simulink model "AN_Simulink_Model_v1_fil"  (R2019b)
settings: Solver=VariableStepAuto  StartTime=0.0  StopTime=testtime  RelTol=1e-3
InitFcn:
  | AN_InitFcn_Callback
StopFcn:
  | AN_StopFcn_Callback
undefined symbols (not defined in the file or in its folder): tdres
libraries: hdlmdlgenlib x193, simulink x4, fillib x1, dspsrcs4 x1
(part 3 of 6)

== system AN_Simulink_Model_v1_fil/Auditory Nerve Model/C2 Wideband Filter/Sum7 ==
  In1 : Inport
  In2 : Inport  Port=2
  Sum7 : Sum  OutDataTypeStr=single  SampleTime=2.08333333333333e-05  SaturateOnIntegerOverflow=on  InputSameDT=on
  Out1 : Outport
  wires:
  Sum7/1 -> Out1/1
  In2/1 -> Sum7/2
  In1/1 -> Sum7/1

== system AN_Simulink_Model_v1_fil/Auditory Nerve Model/C2 Wideband Filter/Sum8 ==
  In1 : Inport
  In2 : Inport  Port=2
  Sum8 : Sum  OutDataTypeStr=single  SampleTime=2.08333333333333e-05  SaturateOnIntegerOverflow=on  InputSameDT=on
  Out1 : Outport
  wires:
  Sum8/1 -> Out1/1
  In2/1 -> Sum8/2
  In1/1 -> Sum8/1

== system AN_Simulink_Model_v1_fil/Auditory Nerve Model/C2 Wideband Filter/Sum9 ==
  In1 : Inport
  In2 : Inport  Port=2
  Sum9 : Sum  OutDataTypeStr=single  SampleTime=2.08333333333333e-05  SaturateOnIntegerOverflow=on  InputSameDT=on
  Out1 : Outport
  wires:
  Sum9/1 -> Out1/1
  In2/1 -> Sum9/2
  In1/1 -> Sum9/1

== system AN_Simulink_Model_v1_fil/Auditory Nerve Model/CP Wideband Gammatone Filter/Calculate wbout ==
  In1 : Inport  OutDataTypeStr=single  PortDimensions=1  SampleTime=2.08333333333333e-05
  In2 : Inport  Port=2  OutDataTypeStr=single  PortDimensions=1  SampleTime=2.08333333333333e-05
  Constant : Constant  Value=single(0.0007758744177408516)  OutDataTypeStr=single  SampleTime=-1
  Constant1 : Constant  Value=single(3)  OutDataTypeStr=single  SampleTime=-1
  Constant3 : Constant  Value=single(1)  OutDataTypeStr=single  SampleTime=-1
  Divide : Subsystem
      mask Display: disp('NFP\nmul');
  Divide1_to_const : Constant  Value=single(0.2)  OutDataTypeStr=single  SampleTime=-1
  Gain : Subsystem
      mask Display: disp('NFP\nmul');
  Gain_const : Constant  Value=single(10000)  OutDataTypeStr=single  SampleTime=-1
  MinMax_stage1_compare : Subsystem
      mask Display: disp('NFP\nrelop');
  MinMax_stage1_switch : Switch  Criteria=u2 ~= 0  Threshold=double(0)  OutDataTypeStr=single  SampleTime=2.08333333333333e-05
  Pow : Subsystem
      mask Display: disp('NFP\nmath2');
  Product : Subsystem
      mask Display: disp('NFP\nmul');
  Product1 : Subsystem
      mask Display: disp('NFP\nmul');
  Out1 : Outport  VectorParamsAs1DForOutWhenUnconnected=off
  wires:
  Gain/1(Out1) -> Product1/1(In1)
  MinMax_stage1_compare/1(Out1) -> MinMax_stage1_switch/2
  Product1/1(Out1) -> Out1/1
  Product/1(Out1) -> Gain/2(In2)
  Pow/1(Out1) -> Product/2(In2)
  Divide/1(Out1) -> Pow/1(In1)
  Gain_const/1 -> Gain/1(In1)
  MinMax_stage1_switch/1 -> Product1/2(In2)
  Divide1_to_const/1 -> MinMax_stage1_switch/1, MinMax_stage1_compare/2(In2)
  Constant3/1 -> MinMax_stage1_switch/3, MinMax_stage1_compare/1(In1)
  Constant1/1 -> Pow/2(In2)
  Constant/1 -> Divide/2(In2)
  In2/1 -> Divide/1(In1)
  In1/1 -> Product/1(In1)

== system AN_Simulink_Model_v1_fil/Auditory Nerve Model/CP Wideband Gammatone Filter/Gain_unaryminus ==
  In1 : Inport
  Gain_unaryminus : UnaryMinus  SampleTime=2.08333333333333e-05
  Out1 : Outport
  wires:
  Gain_unaryminus/1 -> Out1/1
  In1/1 -> Gain_unaryminus/1

== system AN_Simulink_Model_v1_fil/Auditory Nerve Model/CP Wideband Gammatone Filter/MATLAB Function1 ==
  phase : Inport  OutDataTypeStr=single  PortDimensions=1  SampleTime=2.08333333333333e-05
  delta_phase : Inport  Port=2  OutDataTypeStr=single  PortDimensions=1  SampleTime=2.08333333333333e-05
  adder : Subsystem
      mask Display: disp('NFP\nadd');
  adder_outbuff : hdlmdlgenlib/Buffer
      settings: SourceProductName=Simulink  SourceProductBaseCode=SL
  const : Constant  Value=single(6.2831854820251465)  VectorParams1D=off  OutDataTypeStr=single  SampleTime=-1
  const1 : Constant  Value=single(-6.2831854820251465)  VectorParams1D=off  OutDataTypeStr=single  SampleTime=-1
  relop : Subsystem
      mask Display: disp('NFP\nrelop');
  relop_outbuff : hdlmdlgenlib/Buffer
      settings: SourceProductName=Simulink  SourceProductBaseCode=SL
  subtract : Subsystem
      mask Display: disp('NFP\nadd');
  subtract_outbuff : hdlmdlgenlib/Buffer
      settings: SourceProductName=Simulink  SourceProductBaseCode=SL
  switch : Switch  Criteria=u2 ~= 0  Threshold=double(0)  OutDataTypeStr=single  SampleTime=2.08333333333333e-05
  wbphase : Outport  VectorParamsAs1DForOutWhenUnconnected=off
  wires:
  subtract/1(Out1) -> subtract_outbuff/1
  adder/1(Out1) -> adder_outbuff/1
  relop/1(Out1) -> relop_outbuff/1
  const1/1 -> subtract/1(In1)
  const/1 -> adder/2(In2)
  subtract_outbuff/1 -> relop/2(In2)
  adder_outbuff/1 -> switch/1
  relop_outbuff/1 -> switch/2
  switch/1 -> wbphase/1
  delta_phase/1 -> subtract/2(In2)
  phase/1 -> switch/3, relop/1(In1), adder/1(In1)

== system AN_Simulink_Model_v1_fil/Auditory Nerve Model/CP Wideband Gammatone Filter/Product ==
  In1 : Inport
  In2 : Inport  Port=2
  Product : Product  Inputs=**  OutDataTypeStr=single  SampleTime=2.08333333333333e-05
  Out1 : Outport
  wires:
  Product/1 -> Out1/1
  In2/1 -> Product/2
  In1/1 -> Product/1

== system AN_Simulink_Model_v1_fil/Auditory Nerve Model/CP Wideband Gammatone Filter/Product1 ==
  In1 : Inport
  In2 : Inport  Port=2
  Product1 : Product  Inputs=**  OutDataTypeStr=single  SampleTime=2.08333333333333e-05
  Out1 : Outport
  wires:
  Product1/1 -> Out1/1
  In2/1 -> Product1/2
  In1/1 -> Product1/1

== system AN_Simulink_Model_v1_fil/Auditory Nerve Model/CP Wideband Gammatone Filter/Product11 ==
  In1 : Inport
  In2 : Inport  Port=2
  Product11 : Product  Inputs=**  OutDataTypeStr=single  SampleTime=2.08333333333333e-05
  Out1 : Outport
  wires:
  Product11/1 -> Out1/1
  In2/1 -> Product11/2
  In1/1 -> Product11/1

== system AN_Simulink_Model_v1_fil/Auditory Nerve Model/CP Wideband Gammatone Filter/Product12 ==
  In1 : Inport
  In2 : Inport  Port=2
  Product12 : Product  Inputs=**  OutDataTypeStr=single  SampleTime=2.08333333333333e-05
  Out1 : Outport
  wires:
  Product12/1 -> Out1/1
  In2/1 -> Product12/2
  In1/1 -> Product12/1

== system AN_Simulink_Model_v1_fil/Auditory Nerve Model/CP Wideband Gammatone Filter/Product13 ==
  In1 : Inport
  In2 : Inport  Port=2
  Product13 : Product  Inputs=**  OutDataTypeStr=single  SampleTime=2.08333333333333e-05
  Out1 : Outport
  wires:
  Product13/1 -> Out1/1
  In2/1 -> Product13/2
  In1/1 -> Product13/1

== system AN_Simulink_Model_v1_fil/Auditory Nerve Model/CP Wideband Gammatone Filter/Product14 ==
  In1 : Inport
  In2 : Inport  Port=2
  Product14 : Product  Inputs=**  OutDataTypeStr=single  SampleTime=2.08333333333333e-05
  Out1 : Outport
  wires:
  Product14/1 -> Out1/1
  In2/1 -> Product14/2
  In1/1 -> Product14/1

== system AN_Simulink_Model_v1_fil/Auditory Nerve Model/CP Wideband Gammatone Filter/Product1_AC_minus_BD ==
  In1 : Inport
  In2 : Inport  Port=2
  Product1_AC_minus_BD : Sum  Inputs=+-  OutDataTypeStr=single  SampleTime=2.08333333333333e-05  SaturateOnIntegerOverflow=on  InputSameDT=on
  Out1 : Outport
  wires:
  Product1_AC_minus_BD/1 -> Out1/1
  In2/1 -> Product1_AC_minus_BD/2
  In1/1 -> Product1_AC_minus_BD/1

== system AN_Simulink_Model_v1_fil/Auditory Nerve Model/CP Wideband Gammatone Filter/Product1_AD_plus_BC ==
  In1 : Inport
  In2 : Inport  Port=2
  Product1_AD_plus_BC : Sum  OutDataTypeStr=single  SampleTime=2.08333333333333e-05  SaturateOnIntegerOverflow=on  InputSameDT=on
  Out1 : Outport
  wires:
  Product1_AD_plus_BC/1 -> Out1/1
  In2/1 -> Product1_AD_plus_BC/2
  In1/1 -> Product1_AD_plus_BC/1

== system AN_Simulink_Model_v1_fil/Auditory Nerve Model/CP Wideband Gammatone Filter/Sum ==
  In1 : Inport
  In2 : Inport  Port=2
  Sum : Sum  OutDataTypeStr=single  SampleTime=2.08333333333333e-05  SaturateOnIntegerOverflow=on  InputSameDT=on
  Out1 : Outport
  wires:
  Sum/1 -> Out1/1
  In2/1 -> Sum/2
  In1/1 -> Sum/1

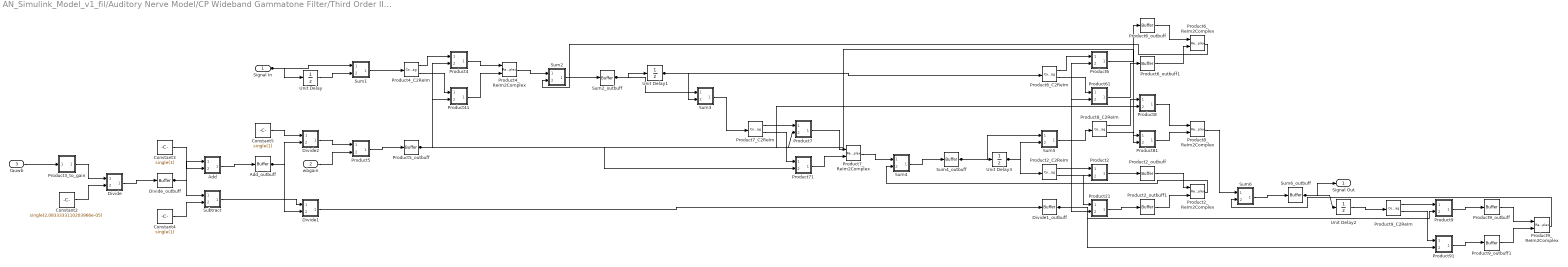
== system AN_Simulink_Model_v1_fil/Auditory Nerve Model/CP Wideband Gammatone Filter/Third Order IIR Filter ==
  Signal In : Inport  OutDataTypeStr=single  PortDimensions=1  SampleTime=2.08333333333333e-05
      settings: SignalType=complex
  wbgain : Inport  Port=2  OutDataTypeStr=single  PortDimensions=1  SampleTime=2.08333333333333e-05
  tauwb : Inport  Port=3  OutDataTypeStr=single  PortDimensions=1  SampleTime=2.08333333333333e-05
  Add : Subsystem
      mask Display: disp('NFP\nadd');
  Add_outbuff : hdlmdlgenlib/Buffer
      settings: SourceProductName=Simulink  SourceProductBaseCode=SL
  Constant2 : Constant  Value=single(2.0833333110203966e-05)  OutDataTypeStr=single  SampleTime=-1
  Constant3 : Constant  Value=single(1)  OutDataTypeStr=single  SampleTime=-1
  Constant4 : Constant  Value=single(1)  OutDataTypeStr=single  SampleTime=-1
  Constant5 : Constant  Value=single(1)  OutDataTypeStr=single  SampleTime=-1
  Divide : Subsystem
      mask Display: disp('NFP\nmul');
  Divide1 : Subsystem
      mask Display: disp('NFP\nmul');
  Divide1_outbuff : hdlmdlgenlib/Buffer
      settings: SourceProductName=Simulink  SourceProductBaseCode=SL
  Divide2 : Subsystem
      mask Display: disp('NFP\nmul');
  Divide_outbuff : hdlmdlgenlib/Buffer
      settings: SourceProductName=Simulink  SourceProductBaseCode=SL
  Product2 : Subsystem
      mask Display: disp('NFP\nmul');
  Product21 : Subsystem
      mask Display: disp('NFP\nmul');
  Product2_C2ReIm : ComplexToRealImag  SampleTime=2.08333333333333e-05
  Product2_ReIm2Complex : RealImagToComplex  SampleTime=2.08333333333333e-05
  Product2_outbuff : hdlmdlgenlib/Buffer
      settings: SourceProductName=Simulink  SourceProductBaseCode=SL
  Product2_outbuff1 : hdlmdlgenlib/Buffer
      settings: SourceProductName=Simulink  SourceProductBaseCode=SL
  Product3_to_gain : Subsystem
      mask Display: disp('NFP\ngain_pow2');
  Product4 : Subsystem
      mask Display: disp('NFP\nmul');
  Product41 : Subsystem
      mask Display: disp('NFP\nmul');
  Product4_C2ReIm : ComplexToRealImag  SampleTime=2.08333333333333e-05
  Product4_ReIm2Complex : RealImagToComplex  SampleTime=2.08333333333333e-05
  Product5 : Subsystem
      mask Display: disp('NFP\nmul');
  Product5_outbuff : hdlmdlgenlib/Buffer
      settings: SourceProductName=Simulink  SourceProductBaseCode=SL
  Product6 : Subsystem
      mask Display: disp('NFP\nmul');
  Product61 : Subsystem
      mask Display: disp('NFP\nmul');
  Product6_C2ReIm : ComplexToRealImag  SampleTime=2.08333333333333e-05
  Product6_ReIm2Complex : RealImagToComplex  SampleTime=2.08333333333333e-05
  Product6_outbuff : hdlmdlgenlib/Buffer
      settings: SourceProductName=Simulink  SourceProductBaseCode=SL
  Product6_outbuff1 : hdlmdlgenlib/Buffer
      settings: SourceProductName=Simulink  SourceProductBaseCode=SL
  Product7 : Subsystem
      mask Display: disp('NFP\nmul');
  Product71 : Subsystem
      mask Display: disp('NFP\nmul');
  Product7_C2ReIm : ComplexToRealImag  SampleTime=2.08333333333333e-05
  Product7_ReIm2Complex : RealImagToComplex  SampleTime=2.08333333333333e-05
  Product8 : Subsystem
      mask Display: disp('NFP\nmul');
  Product81 : Subsystem
      mask Display: disp('NFP\nmul');
  Product8_C2ReIm : ComplexToRealImag  SampleTime=2.08333333333333e-05
  Product8_ReIm2Complex : RealImagToComplex  SampleTime=2.08333333333333e-05
  Product9 : Subsystem
      mask Display: disp('NFP\nmul');
  Product91 : Subsystem
      mask Display: disp('NFP\nmul');
  Product9_C2ReIm : ComplexToRealImag  SampleTime=2.08333333333333e-05
  Product9_ReIm2Complex : RealImagToComplex  SampleTime=2.08333333333333e-05
  Product9_outbuff : hdlmdlgenlib/Buffer
      settings: SourceProductName=Simulink  SourceProductBaseCode=SL
  Product9_outbuff1 : hdlmdlgenlib/Buffer
      settings: SourceProductName=Simulink  SourceProductBaseCode=SL
  Subtract : Subsystem
      mask Display: disp('NFP\nadd');
  Sum1 : Subsystem
      mask Display: disp('NFP\nadd');
  Sum2 : Subsystem
      mask Display: disp('NFP\nadd');
  Sum2_outbuff : hdlmdlgenlib/Buffer
      settings: SourceProductName=Simulink  SourceProductBaseCode=SL
  Sum3 : Subsystem
      mask Display: disp('NFP\nadd');
  Sum4 : Subsystem
      mask Display: disp('NFP\nadd');
  Sum4_outbuff : hdlmdlgenlib/Buffer
      settings: SourceProductName=Simulink  SourceProductBaseCode=SL
  Sum5 : Subsystem
      mask Display: disp('NFP\nadd');
  Sum6 : Subsystem
      mask Display: disp('NFP\nadd');
  Sum6_outbuff : hdlmdlgenlib/Buffer
      settings: SourceProductName=Simulink  SourceProductBaseCode=SL
  Unit Delay{,1..3} (4 alike) : UnitDelay  InitialCondition=single(0)  SampleTime=2.08333333333333e-05
  Signal Out : Outport  VectorParamsAs1DForOutWhenUnconnected=off
  wires:
  Product91/1(Out1) -> Product9_outbuff1/1
  Product9/1(Out1) -> Product9_outbuff/1
  Product81/1(Out1) -> Product8_ReIm2Complex/2
  Product8/1(Out1) -> Product8_ReIm2Complex/1
  Product71/1(Out1) -> Product7_ReIm2Complex/2
  Product7/1(Out1) -> Product7_ReIm2Complex/1
  Product61/1(Out1) -> Product6_outbuff1/1
  Product6/1(Out1) -> Product6_outbuff/1
  Product41/1(Out1) -> Product4_ReIm2Complex/2
  Product4/1(Out1) -> Product4_ReIm2Complex/1
  Product21/1(Out1) -> Product2_outbuff1/1
  Product2/1(Out1) -> Product2_outbuff/1
  Product3_to_gain/1(Out1) -> Divide/1(In1)
  Sum6/1(Out1) -> Sum6_outbuff/1
  Sum5/1(Out1) -> Product8_C2ReIm/1
  Sum4/1(Out1) -> Sum4_outbuff/1
  Sum3/1(Out1) -> Product7_C2ReIm/1
  Sum2/1(Out1) -> Sum2_outbuff/1
  Sum1/1(Out1) -> Product4_C2ReIm/1
  Subtract/1(Out1) -> Divide1/1(In1)
  Product5/1(Out1) -> Product5_outbuff/1
  Divide2/1(Out1) -> Product5/1(In1)
  Divide1/1(Out1) -> Divide1_outbuff/1
  Divide/1(Out1) -> Divide_outbuff/1
  Add/1(Out1) -> Add_outbuff/1
  Product9_outbuff1/1 -> Product9_ReIm2Complex/2
  Product9_outbuff/1 -> Product9_ReIm2Complex/1
  Product9_C2ReIm/2 -> Product91/1(In1)
  Product9_C2ReIm/1 -> Product9/1(In1)
  Product8_C2ReIm/2 -> Product81/1(In1)
  Product8_C2ReIm/1 -> Product8/1(In1)
  Product7_C2ReIm/2 -> Product71/1(In1)
  Product7_C2ReIm/1 -> Product7/1(In1)
  Product6_outbuff1/1 -> Product6_ReIm2Complex/2
  Product6_outbuff/1 -> Product6_ReIm2Complex/1
  Product6_C2ReIm/2 -> Product61/1(In1)
  Product6_C2ReIm/1 -> Product6/1(In1)
  Product4_C2ReIm/2 -> Product41/1(In1)
  Product4_C2ReIm/1 -> Product4/1(In1)
  Product2_outbuff1/1 -> Product2_ReIm2Complex/2
  Product2_outbuff/1 -> Product2_ReIm2Complex/1
  Product2_C2ReIm/2 -> Product21/1(In1)
  Product2_C2ReIm/1 -> Product2/1(In1)
  Unit Delay3/1 -> Product2_C2ReIm/1, Sum5/2(In2)
  Unit Delay2/1 -> Product9_C2ReIm/1
  Unit Delay1/1 -> Product6_C2ReIm/1, Sum3/2(In2)
  Unit Delay/1 -> Sum1/2(In2)
  Sum6_outbuff/1 -> Signal Out/1, Unit Delay2/1
  Sum4_outbuff/1 -> Unit Delay3/1, Sum5/1(In1)
  Sum2_outbuff/1 -> Unit Delay1/1, Sum3/1(In1)
  Product9_ReIm2Complex/1 -> Sum6/2(In2)
  Product8_ReIm2Complex/1 -> Sum6/1(In1)
  Product7_ReIm2Complex/1 -> Sum4/1(In1)
  Product6_ReIm2Complex/1 -> Sum2/2(In2)
  Product5_outbuff/1 -> Product4/2(In2), Product41/2(In2), Product7/2(In2), Product71/2(In2), Product8/2(In2), Product81/2(In2)
  Product4_ReIm2Complex/1 -> Sum2/1(In1)
  Product2_ReIm2Complex/1 -> Sum4/2(In2)
  Divide1_outbuff/1 -> Product2/2(In2), Product21/2(In2), Product6/2(In2), Product61/2(In2), Product9/2(In2), Product91/2(In2)
  Divide_outbuff/1 -> Add/1(In1), Subtract/1(In1)
  Constant5/1 -> Divide2/1(In1)
  Constant4/1 -> Subtract/2(In2)
  Constant3/1 -> Add/2(In2)
  Constant2/1 -> Divide/2(In2)
  Add_outbuff/1 -> Divide1/2(In2), Divide2/2(In2)
  tauwb/1 -> Product3_to_gain/1(In1)
  wbgain/1 -> Product5/2(In2)
  Signal In/1 -> Unit Delay/1, Sum1/1(In1)

== system AN_Simulink_Model_v1_fil/Auditory Nerve Model/CP Wideband Gammatone Filter/Trigonometric Function ==
  In1 : Inport
  Trigonometric Function : Trigonometry  Operator=sincos  SampleTime=2.08333333333333e-05
  Out1 : Outport
  Out2 : Outport  Port=2
  wires:
  Trigonometric Function/2 -> Out2/1
  Trigonometric Function/1 -> Out1/1
  In1/1 -> Trigonometric Function/1

== system AN_Simulink_Model_v1_fil/Auditory Nerve Model/CP Wideband Gammatone Filter/Trigonometric Function1 ==
  In1 : Inport
  Trigonometric Function1 : Trigonometry  Operator=sincos  SampleTime=2.08333333333333e-05
  Out1 : Outport
  Out2 : Outport  Port=2
  wires:
  Trigonometric Function1/2 -> Out2/1
  Trigonometric Function1/1 -> Out1/1
  In1/1 -> Trigonometric Function1/1

== system AN_Simulink_Model_v1_fil/Auditory Nerve Model/Middle Ear Filter/Gain1_unaryminus ==
  In1 : Inport
  Gain1_unaryminus : UnaryMinus  SampleTime=2.08333333333333e-05
  Out1 : Outport
  wires:
  Gain1_unaryminus/1 -> Out1/1
  In1/1 -> Gain1_unaryminus/1

== system AN_Simulink_Model_v1_fil/Auditory Nerve Model/Middle Ear Filter/Gain2_unaryminus ==
  In1 : Inport
  Gain2_unaryminus : UnaryMinus  SampleTime=2.08333333333333e-05
  Out1 : Outport
  wires:
  Gain2_unaryminus/1 -> Out1/1
  In1/1 -> Gain2_unaryminus/1

== system AN_Simulink_Model_v1_fil/Auditory Nerve Model/Middle Ear Filter/Gain3_unaryminus ==
  In1 : Inport
  Gain3_unaryminus : UnaryMinus  SampleTime=2.08333333333333e-05
  Out1 : Outport
  wires:
  Gain3_unaryminus/1 -> Out1/1
  In1/1 -> Gain3_unaryminus/1

== system AN_Simulink_Model_v1_fil/Auditory Nerve Model/Middle Ear Filter/Gain5_unaryminus ==
  In1 : Inport
  Gain5_unaryminus : UnaryMinus  SampleTime=2.08333333333333e-05
  Out1 : Outport
  wires:
  Gain5_unaryminus/1 -> Out1/1
  In1/1 -> Gain5_unaryminus/1

== system AN_Simulink_Model_v1_fil/Auditory Nerve Model/Middle Ear Filter/Gain7_unaryminus ==
  In1 : Inport
  Gain7_unaryminus : UnaryMinus  SampleTime=2.08333333333333e-05
  Out1 : Outport
  wires:
  Gain7_unaryminus/1 -> Out1/1
  In1/1 -> Gain7_unaryminus/1

== system AN_Simulink_Model_v1_fil/Auditory Nerve Model/Middle Ear Filter/Gain8_unaryminus ==
  In1 : Inport
  Gain8_unaryminus : UnaryMinus  SampleTime=2.08333333333333e-05
  Out1 : Outport
  wires:
  Gain8_unaryminus/1 -> Out1/1
  In1/1 -> Gain8_unaryminus/1

== system AN_Simulink_Model_v1_fil/Auditory Nerve Model/Middle Ear Filter/Product ==
  In1 : Inport
  In2 : Inport  Port=2
  Product : Product  Inputs=**  OutDataTypeStr=single  SampleTime=2.08333333333333e-05
  Out1 : Outport
  wires:
  Product/1 -> Out1/1
  In2/1 -> Product/2
  In1/1 -> Product/1

== system AN_Simulink_Model_v1_fil/Auditory Nerve Model/Middle Ear Filter/Product1 ==
  In1 : Inport
  In2 : Inport  Port=2
  Product1 : Product  Inputs=**  OutDataTypeStr=single  SampleTime=2.08333333333333e-05
  Out1 : Outport
  wires:
  Product1/1 -> Out1/1
  In2/1 -> Product1/2
  In1/1 -> Product1/1

== system AN_Simulink_Model_v1_fil/Auditory Nerve Model/Middle Ear Filter/Product10 ==
  In1 : Inport
  In2 : Inport  Port=2
  Product10 : Product  Inputs=**  OutDataTypeStr=single  SampleTime=2.08333333333333e-05
  Out1 : Outport
  wires:
  Product10/1 -> Out1/1
  In2/1 -> Product10/2
  In1/1 -> Product10/1

== system AN_Simulink_Model_v1_fil/Auditory Nerve Model/Middle Ear Filter/Product11 ==
  In1 : Inport
  In2 : Inport  Port=2
  Product11 : Product  Inputs=**  OutDataTypeStr=single  SampleTime=2.08333333333333e-05
  Out1 : Outport
  wires:
  Product11/1 -> Out1/1
  In2/1 -> Product11/2
  In1/1 -> Product11/1

== system AN_Simulink_Model_v1_fil/Auditory Nerve Model/Middle Ear Filter/Product12 ==
  In1 : Inport
  In2 : Inport  Port=2
  Product12 : Product  Inputs=**  OutDataTypeStr=single  SampleTime=2.08333333333333e-05
  Out1 : Outport
  wires:
  Product12/1 -> Out1/1
  In2/1 -> Product12/2
  In1/1 -> Product12/1

== system AN_Simulink_Model_v1_fil/Auditory Nerve Model/Middle Ear Filter/Product13 ==
  In1 : Inport
  In2 : Inport  Port=2
  Product13 : Product  Inputs=**  OutDataTypeStr=single  SampleTime=2.08333333333333e-05
  Out1 : Outport
  wires:
  Product13/1 -> Out1/1
  In2/1 -> Product13/2
  In1/1 -> Product13/1

== system AN_Simulink_Model_v1_fil/Auditory Nerve Model/Middle Ear Filter/Product14 ==
  In1 : Inport
  In2 : Inport  Port=2
  Product14 : Product  Inputs=**  OutDataTypeStr=single  SampleTime=2.08333333333333e-05
  Out1 : Outport
  wires:
  Product14/1 -> Out1/1
  In2/1 -> Product14/2
  In1/1 -> Product14/1

== system AN_Simulink_Model_v1_fil/Auditory Nerve Model/Middle Ear Filter/Product15_to_gain ==
  In1 : Inport
  Product15_to_gain : Gain  Gain=single(0.5)
  Out1 : Outport
  wires:
  Product15_to_gain/1 -> Out1/1
  In1/1 -> Product15_to_gain/1

== system AN_Simulink_Model_v1_fil/Auditory Nerve Model/Middle Ear Filter/Product2 ==
  In1 : Inport
  In2 : Inport  Port=2
  Product2 : Product  Inputs=**  OutDataTypeStr=single  SampleTime=2.08333333333333e-05
  Out1 : Outport
  wires:
  Product2/1 -> Out1/1
  In2/1 -> Product2/2
  In1/1 -> Product2/1

== system AN_Simulink_Model_v1_fil/Auditory Nerve Model/Middle Ear Filter/Product3 ==
  In1 : Inport
  In2 : Inport  Port=2
  Product3 : Product  Inputs=**  OutDataTypeStr=single  SampleTime=2.08333333333333e-05
  Out1 : Outport
  wires:
  Product3/1 -> Out1/1
  In2/1 -> Product3/2
  In1/1 -> Product3/1

== system AN_Simulink_Model_v1_fil/Auditory Nerve Model/Middle Ear Filter/Product4 ==
  In1 : Inport
  In2 : Inport  Port=2
  Product4 : Product  Inputs=**  OutDataTypeStr=single  SampleTime=2.08333333333333e-05
  Out1 : Outport
  wires:
  Product4/1 -> Out1/1
  In2/1 -> Product4/2
  In1/1 -> Product4/1

== system AN_Simulink_Model_v1_fil/Auditory Nerve Model/Middle Ear Filter/Product5 ==
  In1 : Inport
  In2 : Inport  Port=2
  Product5 : Product  Inputs=**  OutDataTypeStr=single  SampleTime=2.08333333333333e-05
  Out1 : Outport
  wires:
  Product5/1 -> Out1/1
  In2/1 -> Product5/2
  In1/1 -> Product5/1

== system AN_Simulink_Model_v1_fil/Auditory Nerve Model/Middle Ear Filter/Product6 ==
  In1 : Inport
  In2 : Inport  Port=2
  Product6 : Product  Inputs=**  OutDataTypeStr=single  SampleTime=2.08333333333333e-05
  Out1 : Outport
  wires:
  Product6/1 -> Out1/1
  In2/1 -> Product6/2
  In1/1 -> Product6/1

== system AN_Simulink_Model_v1_fil/Auditory Nerve Model/Middle Ear Filter/Product7 ==
  In1 : Inport
  In2 : Inport  Port=2
  Product7 : Product  Inputs=**  OutDataTypeStr=single  SampleTime=2.08333333333333e-05
  Out1 : Outport
  wires:
  Product7/1 -> Out1/1
  In2/1 -> Product7/2
  In1/1 -> Product7/1

== system AN_Simulink_Model_v1_fil/Auditory Nerve Model/Middle Ear Filter/Product8 ==
  In1 : Inport
  In2 : Inport  Port=2
  Product8 : Product  Inputs=**  OutDataTypeStr=single  SampleTime=2.08333333333333e-05
  Out1 : Outport
  wires:
  Product8/1 -> Out1/1
  In2/1 -> Product8/2
  In1/1 -> Product8/1

== system AN_Simulink_Model_v1_fil/Auditory Nerve Model/Middle Ear Filter/Product9 ==
  In1 : Inport
  In2 : Inport  Port=2
  Product9 : Product  Inputs=**  OutDataTypeStr=single  SampleTime=2.08333333333333e-05
  Out1 : Outport
  wires:
  Product9/1 -> Out1/1
  In2/1 -> Product9/2
  In1/1 -> Product9/1

== system AN_Simulink_Model_v1_fil/Auditory Nerve Model/Middle Ear Filter/Sum ==
  In1 : Inport
  In2 : Inport  Port=2
  Sum : Sum  OutDataTypeStr=single  SampleTime=2.08333333333333e-05  SaturateOnIntegerOverflow=on  InputSameDT=on
  Out1 : Outport
  wires:
  Sum/1 -> Out1/1
  In2/1 -> Sum/2
  In1/1 -> Sum/1

== system AN_Simulink_Model_v1_fil/Auditory Nerve Model/Middle Ear Filter/Sum1 ==
  In1 : Inport
  In2 : Inport  Port=2
  Sum1 : Sum  OutDataTypeStr=single  SampleTime=2.08333333333333e-05  SaturateOnIntegerOverflow=on  InputSameDT=on
  Out1 : Outport
  wires:
  Sum1/1 -> Out1/1
  In2/1 -> Sum1/2
  In1/1 -> Sum1/1

== system AN_Simulink_Model_v1_fil/Auditory Nerve Model/Middle Ear Filter/Sum10 ==
  In1 : Inport
  In2 : Inport  Port=2
  Sum10 : Sum  OutDataTypeStr=single  SampleTime=2.08333333333333e-05  SaturateOnIntegerOverflow=on  InputSameDT=on
  Out1 : Outport
  wires:
  Sum10/1 -> Out1/1
  In2/1 -> Sum10/2
  In1/1 -> Sum10/1

== system AN_Simulink_Model_v1_fil/Auditory Nerve Model/Middle Ear Filter/Sum11 ==
  In1 : Inport
  In2 : Inport  Port=2
  Sum11 : Sum  OutDataTypeStr=single  SampleTime=2.08333333333333e-05  SaturateOnIntegerOverflow=on  InputSameDT=on
  Out1 : Outport
  wires:
  Sum11/1 -> Out1/1
  In2/1 -> Sum11/2
  In1/1 -> Sum11/1

== system AN_Simulink_Model_v1_fil/Auditory Nerve Model/Middle Ear Filter/Sum2 ==
  In1 : Inport
  In2 : Inport  Port=2
  Sum2 : Sum  OutDataTypeStr=single  SampleTime=2.08333333333333e-05  SaturateOnIntegerOverflow=on  InputSameDT=on
  Out1 : Outport
  wires:
  Sum2/1 -> Out1/1
  In2/1 -> Sum2/2
  In1/1 -> Sum2/1

== system AN_Simulink_Model_v1_fil/Auditory Nerve Model/Middle Ear Filter/Sum3 ==
  In1 : Inport
  In2 : Inport  Port=2
  Sum3 : Sum  OutDataTypeStr=single  SampleTime=2.08333333333333e-05  SaturateOnIntegerOverflow=on  InputSameDT=on
  Out1 : Outport
  wires:
  Sum3/1 -> Out1/1
  In2/1 -> Sum3/2
  In1/1 -> Sum3/1

== system AN_Simulink_Model_v1_fil/Auditory Nerve Model/Middle Ear Filter/Sum4 ==
  In1 : Inport
  In2 : Inport  Port=2
  Sum4 : Sum  OutDataTypeStr=single  SampleTime=2.08333333333333e-05  SaturateOnIntegerOverflow=on  InputSameDT=on
  Out1 : Outport
  wires:
  Sum4/1 -> Out1/1
  In2/1 -> Sum4/2
  In1/1 -> Sum4/1

== system AN_Simulink_Model_v1_fil/Auditory Nerve Model/Middle Ear Filter/Sum5 ==
  In1 : Inport
  In2 : Inport  Port=2
  Sum5 : Sum  OutDataTypeStr=single  SampleTime=2.08333333333333e-05  SaturateOnIntegerOverflow=on  InputSameDT=on
  Out1 : Outport
  wires:
  Sum5/1 -> Out1/1
  In2/1 -> Sum5/2
  In1/1 -> Sum5/1

== system AN_Simulink_Model_v1_fil/Auditory Nerve Model/Middle Ear Filter/Sum6 ==
  In1 : Inport
  In2 : Inport  Port=2
  Sum6 : Sum  OutDataTypeStr=single  SampleTime=2.08333333333333e-05  SaturateOnIntegerOverflow=on  InputSameDT=on
  Out1 : Outport
  wires:
  Sum6/1 -> Out1/1
  In2/1 -> Sum6/2
  In1/1 -> Sum6/1

== system AN_Simulink_Model_v1_fil/Auditory Nerve Model/Middle Ear Filter/Sum7 ==
  In1 : Inport
  In2 : Inport  Port=2
  Sum7 : Sum  OutDataTypeStr=single  SampleTime=2.08333333333333e-05  SaturateOnIntegerOverflow=on  InputSameDT=on
  Out1 : Outport
  wires:
  Sum7/1 -> Out1/1
  In2/1 -> Sum7/2
  In1/1 -> Sum7/1

== system AN_Simulink_Model_v1_fil/Auditory Nerve Model/Middle Ear Filter/Sum8 ==
  In1 : Inport
  In2 : Inport  Port=2
  Sum8 : Sum  OutDataTypeStr=single  SampleTime=2.08333333333333e-05  SaturateOnIntegerOverflow=on  InputSameDT=on
  Out1 : Outport
  wires:
  Sum8/1 -> Out1/1
  In2/1 -> Sum8/2
  In1/1 -> Sum8/1

== system AN_Simulink_Model_v1_fil/Auditory Nerve Model/Middle Ear Filter/Sum9 ==
  In1 : Inport
  In2 : Inport  Port=2
  Sum9 : Sum  OutDataTypeStr=single  SampleTime=2.08333333333333e-05  SaturateOnIntegerOverflow=on  InputSameDT=on
  Out1 : Outport
  wires:
  Sum9/1 -> Out1/1
  In2/1 -> Sum9/2
  In1/1 -> Sum9/1

== system AN_Simulink_Model_v1_fil/Auditory Nerve Model/Subsystem/IHC C1 NL Logarithmic Function ==
  stimulus : Inport  OutDataTypeStr=single  PortDimensions=1  SampleTime=2.08333333333333e-05
  Abs1 : Subsystem
      mask Display: disp('NFP\nabs');
  Add1 : Subsystem
      mask Display: disp('NFP\nadd');
  Compare To Zero1_const : Constant  Value=single(0)  OutDataTypeStr=single  SampleTime=-1
  Compare To Zero1_relop : Subsystem
      mask Display: disp('NFP\nrelop');
  Compare To Zero1_relop_outbuff : hdlmdlgenlib/Buffer
      settings: SourceProductName=Simulink  SourceProductBaseCode=SL
  Constant1 : Constant  Value=single(2000)  OutDataTypeStr=single  SampleTime=-1
  Constant2 : Constant  Value=single(1)  OutDataTypeStr=single  SampleTime=-1
  Constant3 : Constant  Value=single(0.1)  OutDataTypeStr=single  SampleTime=-1
  Log1 : Subsystem
      mask Display: disp('NFP\nmath');
  Product3 : Subsystem
      mask Display: disp('NFP\nmul');
  Product4 : Subsystem
      mask Display: disp('NFP\nmul');
  Product4_outbuff : hdlmdlgenlib/Buffer
      settings: SourceProductName=Simulink  SourceProductBaseCode=SL
  Subsystem1 : Subsystem
  Switch1 : Switch  Criteria=u2 ~= 0  Threshold=double(0)  OutDataTypeStr=single  SampleTime=2.08333333333333e-05
  output : Outport  VectorParamsAs1DForOutWhenUnconnected=off
  wires:
  Product4/1(Out1) -> Product4_outbuff/1
  Product3/1(Out1) -> Add1/1(In1)
  Log1/1(Out1) -> Product4/1(In1)
  Compare To Zero1_relop/1(Out1) -> Compare To Zero1_relop_outbuff/1
  Add1/1(Out1) -> Log1/1(In1)
  Abs1/1(Out1) -> Product3/1(In1)
  Compare To Zero1_const/1 -> Compare To Zero1_relop/2(In2)
  Switch1/1 -> output/1
  Subsystem1/1(Out1) -> Switch1/1
  Product4_outbuff/1 -> Subsystem1/2(In2), Switch1/3
  Constant3/1 -> Product4/2(In2)
  Constant2/1 -> Add1/2(In2)
  Constant1/1 -> Product3/2(In2)
  Compare To Zero1_relop_outbuff/1 -> Subsystem1/3(Enable), Switch1/2
  stimulus/1 -> Subsystem1/1(x), Abs1/1(In1), Compare To Zero1_relop/1(In1)

== system AN_Simulink_Model_v1_fil/Auditory Nerve Model/Subsystem/IHC C2 NL Logarithmic Function ==
  stimulus : Inport  OutDataTypeStr=single  PortDimensions=1  SampleTime=2.08333333333333e-05
  Abs1 : Subsystem
      mask Display: disp('NFP\nabs');
  Add1 : Subsystem
      mask Display: disp('NFP\nadd');
  Compare To Zero1_const : Constant  Value=single(0)  OutDataTypeStr=single  SampleTime=-1
  Compare To Zero1_relop : Subsystem
      mask Display: disp('NFP\nrelop');
  Compare To Zero1_relop_outbuff : hdlmdlgenlib/Buffer
      settings: SourceProductName=Simulink  SourceProductBaseCode=SL
  Constant1 : Constant  Value=single(2000)  OutDataTypeStr=single  SampleTime=-1
  Constant2 : Constant  Value=single(1)  OutDataTypeStr=single  SampleTime=-1
  Constant3 : Constant  Value=single(0.2)  OutDataTypeStr=single  SampleTime=-1
  Log1 : Subsystem
      mask Display: disp('NFP\nmath');
  Product3 : Subsystem
      mask Display: disp('NFP\nmul');
  Product4 : Subsystem
      mask Display: disp('NFP\nmul');
  Product4_outbuff : hdlmdlgenlib/Buffer
      settings: SourceProductName=Simulink  SourceProductBaseCode=SL
  Subsystem1 : Subsystem
  Switch1 : Switch  Criteria=u2 ~= 0  Threshold=double(0)  OutDataTypeStr=single  SampleTime=2.08333333333333e-05
  output : Outport  VectorParamsAs1DForOutWhenUnconnected=off
  wires:
  Product4/1(Out1) -> Product4_outbuff/1
  Product3/1(Out1) -> Add1/1(In1)
  Log1/1(Out1) -> Product4/1(In1)
  Compare To Zero1_relop/1(Out1) -> Compare To Zero1_relop_outbuff/1
  Add1/1(Out1) -> Log1/1(In1)
  Abs1/1(Out1) -> Product3/1(In1)
  Compare To Zero1_const/1 -> Compare To Zero1_relop/2(In2)
  Switch1/1 -> output/1
  Subsystem1/1(Out1) -> Switch1/1
  Product4_outbuff/1 -> Subsystem1/2(In2), Switch1/3
  Constant3/1 -> Product4/2(In2)
  Constant2/1 -> Add1/2(In2)
  Constant1/1 -> Product3/2(In2)
  Compare To Zero1_relop_outbuff/1 -> Subsystem1/3(Enable), Switch1/2
  stimulus/1 -> Subsystem1/1(x), Abs1/1(In1), Compare To Zero1_relop/1(In1)

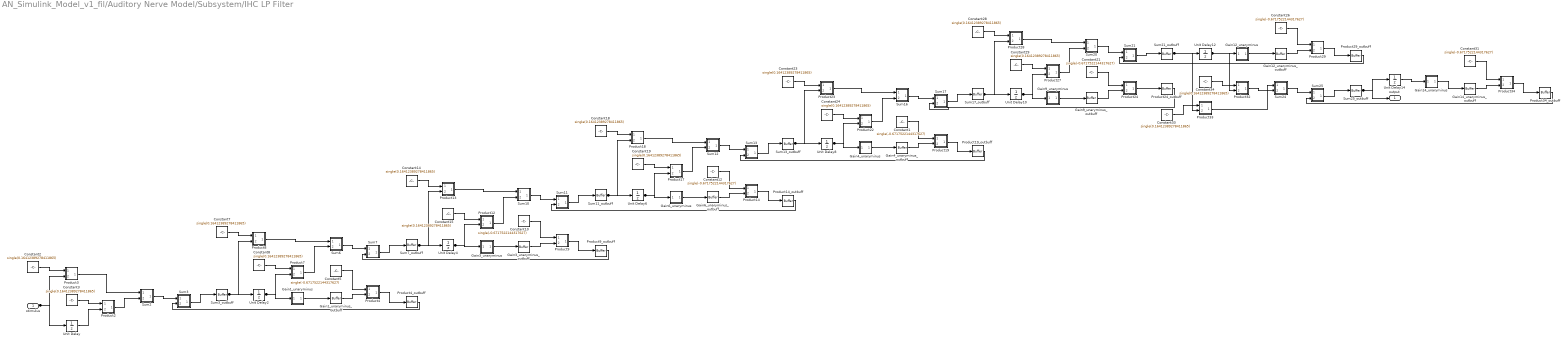
== system AN_Simulink_Model_v1_fil/Auditory Nerve Model/Subsystem/IHC LP Filter ==
  stimulus : Inport  OutDataTypeStr=single  PortDimensions=1  SampleTime=2.08333333333333e-05
  Constant{1,5,10,12,21,26,31} (7 alike) : Constant  Value=single(-0.6717522144317627)  OutDataTypeStr=single  SampleTime=-1
  Constant{2..3,7..8,14..15,18..19,23..24,28..29,33..34} (14 alike) : Constant  Value=single(0.16412389278411865)  OutDataTypeStr=single  SampleTime=-1
  Gain12_unaryminus : Subsystem
      mask Display: disp('NFP\numinus');
  Gain12_unaryminus_outbuff : hdlmdlgenlib/Buffer
      settings: SourceProductName=Simulink  SourceProductBaseCode=SL
  Gain14_unaryminus : Subsystem
      mask Display: disp('NFP\numinus');
  Gain14_unaryminus_outbuff : hdlmdlgenlib/Buffer
      settings: SourceProductName=Simulink  SourceProductBaseCode=SL
  Gain1_unaryminus : Subsystem
      mask Display: disp('NFP\numinus');
  Gain1_unaryminus_outbuff : hdlmdlgenlib/Buffer
      settings: SourceProductName=Simulink  SourceProductBaseCode=SL
  Gain3_unaryminus : Subsystem
      mask Display: disp('NFP\numinus');
  Gain3_unaryminus_outbuff : hdlmdlgenlib/Buffer
      settings: SourceProductName=Simulink  SourceProductBaseCode=SL
  Gain4_unaryminus : Subsystem
      mask Display: disp('NFP\numinus');
  Gain4_unaryminus_outbuff : hdlmdlgenlib/Buffer
      settings: SourceProductName=Simulink  SourceProductBaseCode=SL
  Gain6_unaryminus : Subsystem
      mask Display: disp('NFP\numinus');
  Gain6_unaryminus_outbuff : hdlmdlgenlib/Buffer
      settings: SourceProductName=Simulink  SourceProductBaseCode=SL
  Gain9_unaryminus : Subsystem
      mask Display: disp('NFP\numinus');
  Gain9_unaryminus_outbuff : hdlmdlgenlib/Buffer
      settings: SourceProductName=Simulink  SourceProductBaseCode=SL
  Product12 : Subsystem
      mask Display: disp('NFP\nmul');
  Product13 : Subsystem
      mask Display: disp('NFP\nmul');
  Product14 : Subsystem
      mask Display: disp('NFP\nmul');
  Product14_outbuff : hdlmdlgenlib/Buffer
      settings: SourceProductName=Simulink  SourceProductBaseCode=SL
  Product17 : Subsystem
      mask Display: disp('NFP\nmul');
  Product18 : Subsystem
      mask Display: disp('NFP\nmul');
  Product19 : Subsystem
      mask Display: disp('NFP\nmul');
  Product19_outbuff : hdlmdlgenlib/Buffer
      settings: SourceProductName=Simulink  SourceProductBaseCode=SL
  Product2 : Subsystem
      mask Display: disp('NFP\nmul');
  Product22 : Subsystem
      mask Display: disp('NFP\nmul');
  Product23 : Subsystem
      mask Display: disp('NFP\nmul');
  Product24 : Subsystem
      mask Display: disp('NFP\nmul');
  Product24_outbuff : hdlmdlgenlib/Buffer
      settings: SourceProductName=Simulink  SourceProductBaseCode=SL
  Product27 : Subsystem
      mask Display: disp('NFP\nmul');
  Product28 : Subsystem
      mask Display: disp('NFP\nmul');
  Product29 : Subsystem
      mask Display: disp('NFP\nmul');
  Product29_outbuff : hdlmdlgenlib/Buffer
      settings: SourceProductName=Simulink  SourceProductBaseCode=SL
  Product3 : Subsystem
      mask Display: disp('NFP\nmul');
  Product32 : Subsystem
      mask Display: disp('NFP\nmul');
  Product33 : Subsystem
      mask Display: disp('NFP\nmul');
  Product34 : Subsystem
      mask Display: disp('NFP\nmul');
  Product34_outbuff : hdlmdlgenlib/Buffer
      settings: SourceProductName=Simulink  SourceProductBaseCode=SL
  Product4 : Subsystem
      mask Display: disp('NFP\nmul');
  Product4_outbuff : hdlmdlgenlib/Buffer
      settings: SourceProductName=Simulink  SourceProductBaseCode=SL
  Product7 : Subsystem
      mask Display: disp('NFP\nmul');
  Product8 : Subsystem
      mask Display: disp('NFP\nmul');
  Product9 : Subsystem
      mask Display: disp('NFP\nmul');
  Product9_outbuff : hdlmdlgenlib/Buffer
      settings: SourceProductName=Simulink  SourceProductBaseCode=SL
  Sum10 : Subsystem
      mask Display: disp('NFP\nadd');
  Sum11 : Subsystem
      mask Display: disp('NFP\nadd');
  Sum11_outbuff : hdlmdlgenlib/Buffer
      settings: SourceProductName=Simulink  SourceProductBaseCode=SL
  Sum12 : Subsystem
      mask Display: disp('NFP\nadd');
  Sum13 : Subsystem
      mask Display: disp('NFP\nadd');
  Sum13_outbuff : hdlmdlgenlib/Buffer
      settings: SourceProductName=Simulink  SourceProductBaseCode=SL
  Sum16 : Subsystem
      mask Display: disp('NFP\nadd');
  Sum17 : Subsystem
      mask Display: disp('NFP\nadd');
  Sum17_outbuff : hdlmdlgenlib/Buffer
      settings: SourceProductName=Simulink  SourceProductBaseCode=SL
  Sum2 : Subsystem
      mask Display: disp('NFP\nadd');
  Sum20 : Subsystem
      mask Display: disp('NFP\nadd');
  Sum21 : Subsystem
      mask Display: disp('NFP\nadd');
  Sum21_outbuff : hdlmdlgenlib/Buffer
      settings: SourceProductName=Simulink  SourceProductBaseCode=SL
  Sum24 : Subsystem
      mask Display: disp('NFP\nadd');
  Sum25 : Subsystem
      mask Display: disp('NFP\nadd');
  Sum25_outbuff : hdlmdlgenlib/Buffer
      settings: SourceProductName=Simulink  SourceProductBaseCode=SL
  Sum3 : Subsystem
      mask Display: disp('NFP\nadd');
  Sum3_outbuff : hdlmdlgenlib/Buffer
      settings: SourceProductName=Simulink  SourceProductBaseCode=SL
  Sum6 : Subsystem
      mask Display: disp('NFP\nadd');
  Sum7 : Subsystem
      mask Display: disp('NFP\nadd');
  Sum7_outbuff : hdlmdlgenlib/Buffer
      settings: SourceProductName=Simulink  SourceProductBaseCode=SL
  Unit Delay{,2,4,6,8,10,12,14} (8 alike) : UnitDelay  InitialCondition=single(0)  SampleTime=2.08333333333333e-05
  output : Outport  VectorParamsAs1DForOutWhenUnconnected=off
  wires:
  Sum7/1(Out1) -> Sum7_outbuff/1
  Sum6/1(Out1) -> Sum7/1(In1)
  Sum3/1(Out1) -> Sum3_outbuff/1
  Sum25/1(Out1) -> Sum25_outbuff/1
  Sum24/1(Out1) -> Sum25/1(In1)
  Sum21/1(Out1) -> Sum21_outbuff/1
  Sum20/1(Out1) -> Sum21/1(In1)
  Sum2/1(Out1) -> Sum3/1(In1)
  Sum17/1(Out1) -> Sum17_outbuff/1
  Sum16/1(Out1) -> Sum17/1(In1)
  Sum13/1(Out1) -> Sum13_outbuff/1
  Sum12/1(Out1) -> Sum13/1(In1)
  Sum11/1(Out1) -> Sum11_outbuff/1
  Sum10/1(Out1) -> Sum11/1(In1)
  Product9/1(Out1) -> Product9_outbuff/1
  Product8/1(Out1) -> Sum6/1(In1)
  Product7/1(Out1) -> Sum6/2(In2)
  Product4/1(Out1) -> Product4_outbuff/1
  Product34/1(Out1) -> Product34_outbuff/1
  Product33/1(Out1) -> Sum24/1(In1)
  Product32/1(Out1) -> Sum24/2(In2)
  Product3/1(Out1) -> Sum2/1(In1)
  Product29/1(Out1) -> Product29_outbuff/1
  Product28/1(Out1) -> Sum20/1(In1)
  Product27/1(Out1) -> Sum20/2(In2)
  Product24/1(Out1) -> Product24_outbuff/1
  Product23/1(Out1) -> Sum16/1(In1)
  Product22/1(Out1) -> Sum16/2(In2)
  Product2/1(Out1) -> Sum2/2(In2)
  Product19/1(Out1) -> Product19_outbuff/1
  Product18/1(Out1) -> Sum12/1(In1)
  Product17/1(Out1) -> Sum12/2(In2)
  Product14/1(Out1) -> Product14_outbuff/1
  Product13/1(Out1) -> Sum10/1(In1)
  Product12/1(Out1) -> Sum10/2(In2)
  Gain9_unaryminus/1(Out1) -> Gain9_unaryminus_outbuff/1
  Gain6_unaryminus/1(Out1) -> Gain6_unaryminus_outbuff/1
  Gain4_unaryminus/1(Out1) -> Gain4_unaryminus_outbuff/1
  Gain3_unaryminus/1(Out1) -> Gain3_unaryminus_outbuff/1
  Gain14_unaryminus/1(Out1) -> Gain14_unaryminus_outbuff/1
  Gain12_unaryminus/1(Out1) -> Gain12_unaryminus_outbuff/1
  Gain1_unaryminus/1(Out1) -> Gain1_unaryminus_outbuff/1
  Unit Delay8/1 -> Gain4_unaryminus/1(In1), Product22/2(In2)
  Unit Delay6/1 -> Gain6_unaryminus/1(In1), Product17/2(In2)
  Unit Delay4/1 -> Gain3_unaryminus/1(In1), Product12/2(In2)
  Unit Delay2/1 -> Gain1_unaryminus/1(In1), Product7/2(In2)
  Unit Delay14/1 -> Gain14_unaryminus/1(In1)
  Unit Delay12/1 -> Gain12_unaryminus/1(In1), Product32/2(In2)
  Unit Delay10/1 -> Gain9_unaryminus/1(In1), Product27/2(In2)
  Unit Delay/1 -> Product2/2(In2)
  Sum7_outbuff/1 -> Unit Delay4/1, Product13/2(In2)
  Sum3_outbuff/1 -> Unit Delay2/1, Product8/2(In2)
  Sum25_outbuff/1 -> output/1, Unit Delay14/1
  Sum21_outbuff/1 -> Unit Delay12/1, Product33/2(In2)
  Sum17_outbuff/1 -> Unit Delay10/1, Product28/2(In2)
  Sum13_outbuff/1 -> Unit Delay8/1, Product23/2(In2)
  Sum11_outbuff/1 -> Unit Delay6/1, Product18/2(In2)
  Product9_outbuff/1 -> Sum7/2(In2)
  Product4_outbuff/1 -> Sum3/2(In2)
  Product34_outbuff/1 -> Sum25/2(In2)
  Product29_outbuff/1 -> Sum21/2(In2)
  Product24_outbuff/1 -> Sum17/2(In2)
  Product19_outbuff/1 -> Sum13/2(In2)
  Product14_outbuff/1 -> Sum11/2(In2)
  Gain9_unaryminus_outbuff/1 -> Product24/2(In2)
  Gain6_unaryminus_outbuff/1 -> Product14/2(In2)
  Gain4_unaryminus_outbuff/1 -> Product19/2(In2)
  Gain3_unaryminus_outbuff/1 -> Product9/2(In2)
  Gain14_unaryminus_outbuff/1 -> Product34/2(In2)
  Gain12_unaryminus_outbuff/1 -> Product29/2(In2)
  Gain1_unaryminus_outbuff/1 -> Product4/2(In2)
  Constant8/1 -> Product7/1(In1)
  Constant7/1 -> Product8/1(In1)
  Constant5/1 -> Product4/1(In1)
  Constant34/1 -> Product32/1(In1)
  Constant33/1 -> Product33/1(In1)
  Constant31/1 -> Product34/1(In1)
  Constant3/1 -> Product2/1(In1)
  Constant29/1 -> Product27/1(In1)
  Constant28/1 -> Product28/1(In1)
  Constant26/1 -> Product29/1(In1)
  Constant24/1 -> Product22/1(In1)
  Constant23/1 -> Product23/1(In1)
  Constant21/1 -> Product24/1(In1)
  Constant2/1 -> Product3/1(In1)
  Constant19/1 -> Product17/1(In1)
  Constant18/1 -> Product18/1(In1)
  Constant15/1 -> Product12/1(In1)
  Constant14/1 -> Product13/1(In1)
  Constant12/1 -> Product14/1(In1)
  Constant10/1 -> Product9/1(In1)
  Constant1/1 -> Product19/1(In1)
  stimulus/1 -> Unit Delay/1, Product3/2(In2)

== system AN_Simulink_Model_v1_fil/Auditory Nerve Model/Subsystem/Sum1 ==
  In1 : Inport
  In2 : Inport  Port=2
  Sum1 : Sum  OutDataTypeStr=single  SampleTime=2.08333333333333e-05  SaturateOnIntegerOverflow=on  InputSameDT=on
  Out1 : Outport
  wires:
  Sum1/1 -> Out1/1
  In2/1 -> Sum1/2
  In1/1 -> Sum1/1

== system AN_Simulink_Model_v1_fil/Auditory Nerve Model/Subsystem1/Calculate tauc1 ==
  In1 : Inport  OutDataTypeStr=single  PortDimensions=1  SampleTime=2.08333333333333e-05
  Add : Subsystem
      mask Display: disp('NFP\nadd');
  Constant1 : Constant  Value=single(0.00046310402103699744)  OutDataTypeStr=single  SampleTime=-1
  Constant2 : Constant  Value=single(0.00046310402103699744)  OutDataTypeStr=single  SampleTime=-1
  Product_to_gain : Subsystem
      mask Display: disp('NFP\ngain_pow2');
  Subtract : Subsystem
      mask Display: disp('NFP\nadd');
  Out1 : Outport  VectorParamsAs1DForOutWhenUnconnected=off
  wires:
  Product_to_gain/1(Out1) -> Add/1(In1)
  Subtract/1(Out1) -> Product_to_gain/1(In1)
  Add/1(Out1) -> Out1/1
  Constant2/1 -> Add/2(In2)
  Constant1/1 -> Subtract/2(In2)
  In1/1 -> Subtract/1(In1)

== system AN_Simulink_Model_v1_fil/Auditory Nerve Model/Subsystem1/NL After OHC Function ==
  stimulus : Inport  OutDataTypeStr=single  PortDimensions=1  SampleTime=2.08333333333333e-05
  Abs : Subsystem
      mask Display: disp('NFP\nabs');
  Add3 : Subsystem
      mask Display: disp('NFP\nadd');
  Constant12 : Constant  Value=single(0.05)  OutDataTypeStr=single  SampleTime=-1
  Constant15 : Constant  Value=single(0.003011211520060897)  OutDataTypeStr=single  SampleTime=-1
  Constant5 : Constant  Value=single(0.146789088845253)  OutDataTypeStr=single  SampleTime=-1
  Divide1 : Subsystem
      mask Display: disp('NFP\nmul');
  Exp : Subsystem
      mask Display: disp('NFP\nmath');
  Gain2_unaryminus : Subsystem
      mask Display: disp('NFP\numinus');
  Product3 : Subsystem
      mask Display: disp('NFP\nmul');
  Product4 : Subsystem
      mask Display: disp('NFP\nmul');
  Product4_outbuff : hdlmdlgenlib/Buffer
      settings: SourceProductName=Simulink  SourceProductBaseCode=SL
  Saturation_LowerConst : Constant  Value=single(0.00046310402103699744)  OutDataTypeStr=single  SampleTime=-1
  Saturation_LowerRelop : Subsystem
      mask Display: disp('NFP\nrelop');
  Saturation_Switch1 : Switch  Criteria=u2 ~= 0  Threshold=double(0)  OutDataTypeStr=single  SampleTime=2.08333333333333e-05
  Saturation_Switch2 : Switch  Criteria=u2 ~= 0  Threshold=double(0)  OutDataTypeStr=single  SampleTime=2.08333333333333e-05
  Saturation_UpperConst : Constant  Value=single(0.003011211520060897)  OutDataTypeStr=single  SampleTime=-1
  Saturation_UpperRelop : Subsystem
      mask Display: disp('NFP\nrelop');
  Subtract4_to_const : Constant  Value=single(0.95)  OutDataTypeStr=single  SampleTime=-1
  output : Outport  VectorParamsAs1DForOutWhenUnconnected=off
  wires:
  Saturation_LowerRelop/1(Out1) -> Saturation_Switch2/2
  Saturation_UpperRelop/1(Out1) -> Saturation_Switch1/2
  Product4/1(Out1) -> Product4_outbuff/1
  Product3/1(Out1) -> Add3/2(In2)
  Exp/1(Out1) -> Product3/2(In2)
  Divide1/1(Out1) -> Gain2_unaryminus/1(In1)
  Add3/1(Out1) -> Product4/2(In2)
  Abs/1(Out1) -> Divide1/1(In1)
  Gain2_unaryminus/1(Out1) -> Exp/1(In1)
  Saturation_Switch1/1 -> Saturation_Switch2/3
  Saturation_UpperConst/1 -> Saturation_Switch2/1, Saturation_LowerRelop/2(In2)
  Saturation_LowerConst/1 -> Saturation_Switch1/1, Saturation_UpperRelop/2(In2)
  Subtract4_to_const/1 -> Product3/1(In1)
  Saturation_Switch2/1 -> output/1
  Product4_outbuff/1 -> Saturation_Switch1/3, Saturation_UpperRelop/1(In1), Saturation_LowerRelop/1(In1)
  Constant5/1 -> Divide1/2(In2)
  Constant15/1 -> Product4/1(In1)
  Constant12/1 -> Add3/1(In1)
  stimulus/1 -> Abs/1(In1)

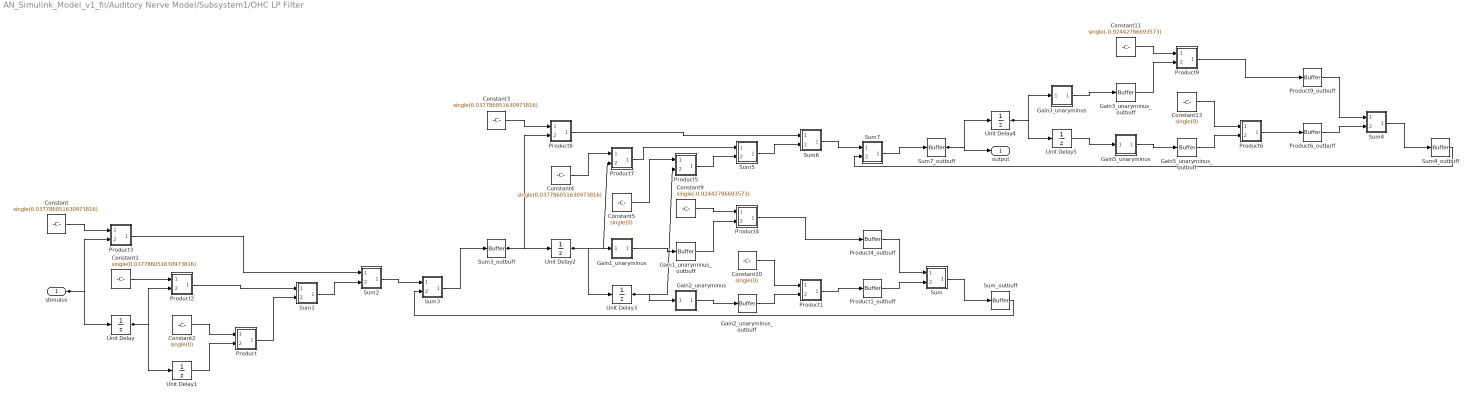
== system AN_Simulink_Model_v1_fil/Auditory Nerve Model/Subsystem1/OHC LP Filter ==
  stimulus : Inport  OutDataTypeStr=single  PortDimensions=1  SampleTime=2.08333333333333e-05
  Constant{,1,3..4} (4 alike) : Constant  Value=single(0.037786051630973816)  OutDataTypeStr=single  SampleTime=-1
  Constant{2,5,10,13} (4 alike) : Constant  Value=single(0)  OutDataTypeStr=single  SampleTime=-1
  Constant11 : Constant  Value=single(-0.92442786693573)  OutDataTypeStr=single  SampleTime=-1
  Constant9 : Constant  Value=single(-0.92442786693573)  OutDataTypeStr=single  SampleTime=-1
  Gain1_unaryminus : Subsystem
      mask Display: disp('NFP\numinus');
  Gain1_unaryminus_outbuff : hdlmdlgenlib/Buffer
      settings: SourceProductName=Simulink  SourceProductBaseCode=SL
  Gain2_unaryminus : Subsystem
      mask Display: disp('NFP\numinus');
  Gain2_unaryminus_outbuff : hdlmdlgenlib/Buffer
      settings: SourceProductName=Simulink  SourceProductBaseCode=SL
  Gain3_unaryminus : Subsystem
      mask Display: disp('NFP\numinus');
  Gain3_unaryminus_outbuff : hdlmdlgenlib/Buffer
      settings: SourceProductName=Simulink  SourceProductBaseCode=SL
  Gain5_unaryminus : Subsystem
      mask Display: disp('NFP\numinus');
  Gain5_unaryminus_outbuff : hdlmdlgenlib/Buffer
      settings: SourceProductName=Simulink  SourceProductBaseCode=SL
  Product : Subsystem
      mask Display: disp('NFP\nmul');
  Product1 : Subsystem
      mask Display: disp('NFP\nmul');
  Product1_outbuff : hdlmdlgenlib/Buffer
      settings: SourceProductName=Simulink  SourceProductBaseCode=SL
  Product2 : Subsystem
      mask Display: disp('NFP\nmul');
  Product3 : Subsystem
      mask Display: disp('NFP\nmul');
  Product4 : Subsystem
      mask Display: disp('NFP\nmul');
  Product4_outbuff : hdlmdlgenlib/Buffer
      settings: SourceProductName=Simulink  SourceProductBaseCode=SL
  Product5 : Subsystem
      mask Display: disp('NFP\nmul');
  Product6 : Subsystem
      mask Display: disp('NFP\nmul');
  Product6_outbuff : hdlmdlgenlib/Buffer
      settings: SourceProductName=Simulink  SourceProductBaseCode=SL
  Product7 : Subsystem
      mask Display: disp('NFP\nmul');
  Product8 : Subsystem
      mask Display: disp('NFP\nmul');
  Product9 : Subsystem
      mask Display: disp('NFP\nmul');
  Product9_outbuff : hdlmdlgenlib/Buffer
      settings: SourceProductName=Simulink  SourceProductBaseCode=SL
  Sum : Subsystem
      mask Display: disp('NFP\nadd');
  Sum1 : Subsystem
      mask Display: disp('NFP\nadd');
  Sum2 : Subsystem
      mask Display: disp('NFP\nadd');
  Sum3 : Subsystem
      mask Display: disp('NFP\nadd');
  Sum3_outbuff : hdlmdlgenlib/Buffer
      settings: SourceProductName=Simulink  SourceProductBaseCode=SL
  Sum4 : Subsystem
      mask Display: disp('NFP\nadd');
  Sum4_outbuff : hdlmdlgenlib/Buffer
      settings: SourceProductName=Simulink  SourceProductBaseCode=SL
  Sum5 : Subsystem
      mask Display: disp('NFP\nadd');
  Sum6 : Subsystem
      mask Display: disp('NFP\nadd');
  Sum7 : Subsystem
      mask Display: disp('NFP\nadd');
  Sum7_outbuff : hdlmdlgenlib/Buffer
      settings: SourceProductName=Simulink  SourceProductBaseCode=SL
  Sum_outbuff : hdlmdlgenlib/Buffer
      settings: SourceProductName=Simulink  SourceProductBaseCode=SL
  Unit Delay{,1..5} (6 alike) : UnitDelay  InitialCondition=single(0)  SampleTime=2.08333333333333e-05
  output : Outport  VectorParamsAs1DForOutWhenUnconnected=off
  wires:
  Sum7/1(Out1) -> Sum7_outbuff/1
  Sum6/1(Out1) -> Sum7/1(In1)
  Sum5/1(Out1) -> Sum6/2(In2)
  Sum4/1(Out1) -> Sum4_outbuff/1
  Sum3/1(Out1) -> Sum3_outbuff/1
  Sum2/1(Out1) -> Sum3/1(In1)
  Sum1/1(Out1) -> Sum2/2(In2)
  Sum/1(Out1) -> Sum_outbuff/1
  Product9/1(Out1) -> Product9_outbuff/1
  Product8/1(Out1) -> Sum6/1(In1)
  Product7/1(Out1) -> Sum5/1(In1)
  Product6/1(Out1) -> Product6_outbuff/1
  Product5/1(Out1) -> Sum5/2(In2)
  Product4/1(Out1) -> Product4_outbuff/1
  Product3/1(Out1) -> Sum2/1(In1)
  Product2/1(Out1) -> Sum1/1(In1)
  Product1/1(Out1) -> Product1_outbuff/1
  Product/1(Out1) -> Sum1/2(In2)
  Gain5_unaryminus/1(Out1) -> Gain5_unaryminus_outbuff/1
  Gain3_unaryminus/1(Out1) -> Gain3_unaryminus_outbuff/1
  Gain2_unaryminus/1(Out1) -> Gain2_unaryminus_outbuff/1
  Gain1_unaryminus/1(Out1) -> Gain1_unaryminus_outbuff/1
  Unit Delay5/1 -> Gain5_unaryminus/1(In1)
  Unit Delay4/1 -> Unit Delay5/1, Gain3_unaryminus/1(In1)
  Unit Delay3/1 -> Gain2_unaryminus/1(In1), Product5/2(In2)
  Unit Delay2/1 -> Unit Delay3/1, Gain1_unaryminus/1(In1), Product7/2(In2)
  Unit Delay1/1 -> Product/2(In2)
  Unit Delay/1 -> Unit Delay1/1, Product2/2(In2)
  Sum7_outbuff/1 -> output/1, Unit Delay4/1
  Sum4_outbuff/1 -> Sum7/2(In2)
  Sum3_outbuff/1 -> Unit Delay2/1, Product8/2(In2)
  Sum_outbuff/1 -> Sum3/2(In2)
  Product9_outbuff/1 -> Sum4/1(In1)
  Product6_outbuff/1 -> Sum4/2(In2)
  Product4_outbuff/1 -> Sum/1(In1)
  Product1_outbuff/1 -> Sum/2(In2)
  Gain5_unaryminus_outbuff/1 -> Product6/2(In2)
  Gain3_unaryminus_outbuff/1 -> Product9/2(In2)
  Gain2_unaryminus_outbuff/1 -> Product1/2(In2)
  Gain1_unaryminus_outbuff/1 -> Product4/2(In2)
  Constant9/1 -> Product4/1(In1)
  Constant5/1 -> Product5/1(In1)
  Constant4/1 -> Product7/1(In1)
  Constant3/1 -> Product8/1(In1)
  Constant2/1 -> Product/1(In1)
  Constant13/1 -> Product6/1(In1)
  Constant11/1 -> Product9/1(In1)
  Constant10/1 -> Product1/1(In1)
  Constant1/1 -> Product2/1(In1)
  Constant/1 -> Product3/1(In1)
  stimulus/1 -> Unit Delay/1, Product3/2(In2)
